simulink model "modor_modeli_z_domain"  (R2024a)
settings: Solver=ode45  StartTime=0.0  StopTime=20  FixedStep=0.01  RelTol=1e-3
values from neighbouring files (symbols this model uses):
  B = 0.0001    [Motor_verileri.m]    (also in deneme1_proje_z.m)
  J = 0.004    [Motor_verileri.m]    (also in deneme1_proje_z.m = 0.0001)
  Kd = 0.000033    (= 3.3e-05)    [Motor_verileri.m]
  Ke = 0.12    [Motor_verileri.m]    (also in deneme1_proje_z.m = 0.05)
  Ki = 2.43    [Motor_verileri.m]
  Ki_tasarim = (q1 + q0) / Ts    [os_zeta.m]
  Kp = 0.0114    [Motor_verileri.m]
  Kp_tasarim = -q0    [os_zeta.m]
  Kt = 0.12    [Motor_verileri.m]    (also in deneme1_proje_z.m = 0.05)
  L = 0.00005    (= 5e-05)    [Motor_verileri.m]    (also in deneme1_proje_z.m)
  R = 0.017    [Motor_verileri.m]    (also in deneme1_proje_z.m)
undefined symbols (not defined in the file or in its folder): DiscIntNeverNeededParam
libraries: simulink x2, slpidlib x1
settings Model: Creator=user  LastModifiedBy=user

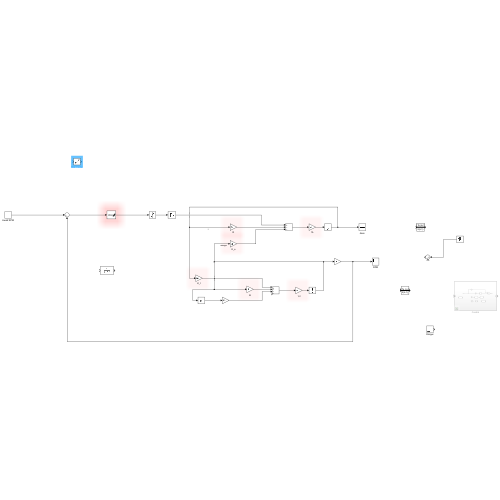
[thumbnail: Simulink's stored preview of the top-level diagram]
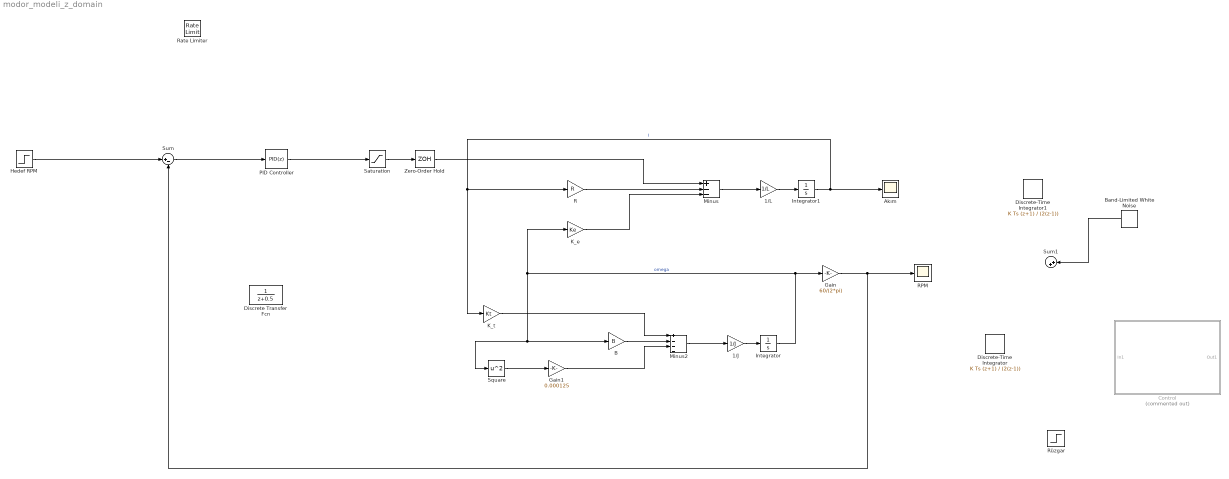
== system modor_modeli_z_domain ==
  1/J : Gain  Gain=1/J
  1/L : Gain  Gain=1/L
  Akım : Scope
  B : Gain  Gain=B
  Band-Limited White Noise : simulink/Sources/Band-Limited White Noise  Cov=[0.0001]  Ts=0.01  seed=[23341]
  Control : Subsystem  Commented=on
  Discrete Transfer Fcn : DiscreteTransferFcn
  Discrete-Time Integrator : DiscreteIntegrator  IntegratorMethod=Integration: Trapezoidal  SampleTime=0.01  ICPrevOutput=DiscIntNeverNeededParam  ICPrevScaledInput=DiscIntNeverNeededParam
  Discrete-Time Integrator1 : DiscreteIntegrator  IntegratorMethod=Integration: Trapezoidal  SampleTime=0.01  ICPrevOutput=DiscIntNeverNeededParam  ICPrevScaledInput=DiscIntNeverNeededParam
  Gain : Gain  Gain=60/(2*pi)
  Gain1 : Gain  Gain=0.000125
  Hedef RPM : Step  Time=0.1  After=500  SampleTime=0.01
  Integrator : Integrator
  Integrator1 : Integrator
  K_e : Gain  Gain=Ke
  K_t : Gain  Gain=Kt
  Minus : Sum  Inputs=+--
  Minus2 : Sum  Inputs=+---
  PID Controller : slpidlib/PID Controller  Controller=PID  Form=Parallel  TimeDomain=Discrete-time  UseExternalTs=off  SampleTime=0.01  IntegratorMethod=Forward Euler  FilterMethod=Forward Euler  ControllerParametersSource=internal  P=Kp_tasarim  I=Ki_tasarim  UseKiTs=off  D=0  UseExternalDerivativeSource=off  N=100  UseFilter=on  TunerSelectOption=Transfer Function Based (PID Tuner App)  InitialConditionSource=internal  InitialConditionForIntegrator=0  InitialConditionForFilter=0  DifferentiatorICPrevScaledInput=0  ExternalReset=none  TrackingMode=off  Kt=1  LimitOutput=on  SatLimitsSource=internal  UpperSaturationLimit=60  LowerSaturationLimit=0  LinearizeAsGain=on  AntiWindupMode=clamping  Kb=1  LimitIntegrator=on  UpperIntegratorSaturationLimit=60  LowerIntegratorSaturationLimit=0  POutMin=[]  POutMax=[]  IOutMin=[]  IOutMax=[]  DOutMin=[]  DOutMax=[]  NOutMin=[]  NOutMax=[]  SumOutMin=[]  SumOutMax=[]  SaturationOutMin=[]  SaturationOutMax=[]  PParamMin=[]  PParamMax=[]  IParamMin=[]  IParamMax=[]  DParamMin=[]  DParamMax=[]  NParamMin=[]  NParamMax=[]  KbParamMin=[]  KbParamMax=[]  KtParamMin=[]  KtParamMax=[]  KbOutMin=[]  KbOutMax=[]  KtOutMin=[]  KtOutMax=[]  IntegratorOutMin=[]  IntegratorOutMax=[]  FilterOutMin=[]  FilterOutMax=[]  SumI1OutMin=[]  SumI1OutMax=[]  SumI2OutMin=[]  SumI2OutMax=[]  SumI3OutMin=[]  SumI3OutMax=[]  SumI4OutMin=[]  SumI4OutMax=[]  SumDOutMin=[]  SumDOutMax=[]  DifferentiatorOutMin=[]  DifferentiatorOutMax=[]  FilterDiffOutCoefMin=[]  FilterDiffOutCoefMax=[]  ReciprocalOutMin=[]  ReciprocalOutMax=[]  SumDenOutMin=[]  SumDenOutMax=[]  SumNumOutMin=[]  SumNumOutMax=[]  DivideOutMin=[]  DivideOutMax=[]  UdiffTsProdOutMin=[]  UdiffTsProdOutMax=[]  NTsProdOutMin=[]  NTsProdOutMax=[]  UintegralTsProdOutMin=[]  UintegralTsProdOutMax=[]  UngainTsProdOutMin=[]  UngainTsProdOutMax=[]  ClampingZeroOutDataTypeStr=Inherit: Inherit via back propagation  ClampingZeroOutMin=[]  ClampingZeroOutMax=[]  FilterDenConstantOutDataTypeStr=Inherit: Inherit via back propagation  FilterDenConstantOutMin=[]  FilterDenConstantOutMax=[]  PCopyOutDataTypeStr=Inherit: Inherit via back propagation  PCopyOutMin=[]  PCopyOutMax=[]  NCopyOutDataTypeStr=Inherit: Inherit via back propagation  NCopyOutMin=[]  NCopyOutMax=[]  IntegratorContinuousStateAttributes=''  IntegratorStateMustResolveToSignalObject=off  IntegratorRTWStateStorageClass=Auto  FilterContinuousStateAttributes=''  FilterStateMustResolveToSignalObject=off  FilterRTWStateStorageClass=Auto  ParallelPVariant=InternalParameters  IdealPVariant=Disabled  IVariant=InternalParameters  DVariant=InternalParameters  IntegratorVariant=Discrete  SatVariant=Enabled  AWVariant=DiscClampingParallel  PCopyVariant=Disabled  TRVariant=Disabled  FdbkBlocksVariant=Forward  IdealPFdbkVariant=Disabled  SatFdbkVariant=Disabled  DerivativeFilterVariant=ForwardEulerFilter  NVariant=InternalParameters  NCopyVariant=Disabled  FilterICVariant=InternalICsFilter  IntegratorICVariant=InternalICs  ExternalResetVariant=Disabled  TRSumVariant=Passthrough  SumFdbkVariant=Disabled  SumVariant=Sum_PID  TsampFilterVariant=InternalTs  TsampNgainVariant=Passthrough  TsampIntegralVariant=Disabled_SignalSpec  ExternalSaturationOutDataTypeStr=Inherit: Same as second input  DerivativeSourceVariant=ErrorSignal
  R : Gain  Gain=R
  RPM : Scope
  Rate Limiter : RateLimiter  RisingSlewLimit=1000  FallingSlewLimit=-1000  SampleTimeMode=inherited
  Rüzgar : Step  Time=0.5  After=5  SampleTime=0
  Saturation : Saturate  UpperLimit=60  LowerLimit=0
  Square : Math  Operator=square
  Sum : Sum  Inputs=|+-
  Sum1 : Sum  Inputs=|++
  Zero-Order Hold : ZeroOrderHold  SampleTime=0.01
  wires:
  Band-Limited White Noise/1 -> Sum1/1
  R/1 -> Minus/2
  Minus/1 -> 1/L/1
  Square/1 -> Gain1/1
  K_e/1 -> Minus/3
  Integrator/1 -> K_e/1, Square/1, B/1, Gain/1  "omega"
  Gain1/1 -> Minus2/3
  Minus2/1 -> 1/J/1
  Integrator1/1 -> K_t/1, R/1, Akım/1  "I"
  1/J/1 -> Integrator/1
  K_t/1 -> Minus2/1
  B/1 -> Minus2/2
  1/L/1 -> Integrator1/1
  Zero-Order Hold/1 -> Minus/1
  Hedef RPM/1 -> Sum/1
  Saturation/1 -> Zero-Order Hold/1
  Gain/1 -> Sum/2, RPM/1
  PID Controller/1 -> Saturation/1
  Sum/1 -> PID Controller/1

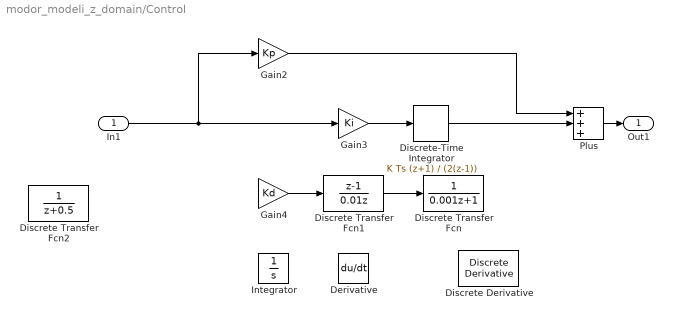
== system modor_modeli_z_domain/Control ==
  In1 : Inport
  Derivative : Derivative
  Discrete Transfer Fcn : DiscreteTransferFcn  Denominator=[0.001 1]
  Discrete Transfer Fcn1 : DiscreteTransferFcn  Numerator=[1 -1]  Denominator=[0.01 0]
  Discrete Transfer Fcn2 : DiscreteTransferFcn
  Discrete Derivative : simulink/Discrete/Discrete Derivative  gainval=1.0  ICPrevScaledInput=0.0  OutMin=[]  OutMax=[]  OutDataType=fixdt(1, 16)  OutScaling=2^-10  DoSatur=off
  Discrete-Time Integrator : DiscreteIntegrator  IntegratorMethod=Integration: Trapezoidal  SampleTime=0.01  LimitOutput=on  UpperSaturationLimit=60  LowerSaturationLimit=0  ICPrevOutput=DiscIntNeverNeededParam  ICPrevScaledInput=DiscIntNeverNeededParam
  Gain2 : Gain  Gain=Kp
  Gain3 : Gain  Gain=Ki
  Gain4 : Gain  Gain=Kd
  Integrator : Integrator  LimitOutput=on  UpperSaturationLimit=60  LowerSaturationLimit=0
  Plus : Sum  Inputs=+++
  Out1 : Outport
  wires:
  In1/1 -> Gain2/1, Gain3/1
  Gain4/1 -> Discrete Transfer Fcn1/1
  Gain2/1 -> Plus/1
  Gain3/1 -> Discrete-Time Integrator/1
  Plus/1 -> Out1/1
  Discrete-Time Integrator/1 -> Plus/2
  Discrete Transfer Fcn1/1 -> Discrete Transfer Fcn/1
